simulink model "speed_controller_Harness1"  (R2020b)
settings: Solver=FixedStepDiscrete  StartTime=0.0  StopTime=500  FixedStep=double(Ts)  RelTol=1e-3
settings Model: DataDictionary=speed_controller.sldd  Creator=Dmitry  LastModifiedBy=Dmitry

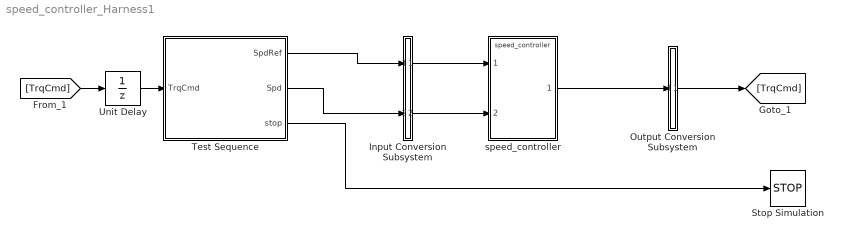
== system speed_controller_Harness1 ==
  Input Conversion Subsystem : Subsystem  Tag=__SLT_ICS__  Description=|
      | Signal spec.
      | and routing
      settings: AttributesFormatString=%<Description>
  Output Conversion Subsystem : Subsystem  Tag=__SLT_OCS__  Description=|
      | Signal spec.
      | and routing
      settings: AttributesFormatString=%<Description>
  Stop Simulation : Stop
  Test Sequence : Test Sequence  TreatAsAtomicUnit=on
  Unit Delay : UnitDelay  SampleTime=-1  HasFrameUpgradeWarning=on
  speed_controller : ModelReference  ModelNameDialog=speed_controller  SimulationMode=Normal  ModelReferenceVersion=1.4
  wires:
  Test Sequence/1(SpdRef) -> Input Conversion Subsystem/1(Inport_1)
  Test Sequence/2(Spd) -> Input Conversion Subsystem/2(Inport_2)
  [TrqCmd] -> Unit Delay/1
  Output Conversion Subsystem/1(Outport_1) -> [TrqCmd]
  Input Conversion Subsystem/1(Outport_1) -> speed_controller/1
  Input Conversion Subsystem/2(Outport_2) -> speed_controller/2
  speed_controller/1 -> Output Conversion Subsystem/1(Inport_1)
  Unit Delay/1 -> Test Sequence/1(TrqCmd)
  Test Sequence/3(stop) -> Stop Simulation/1

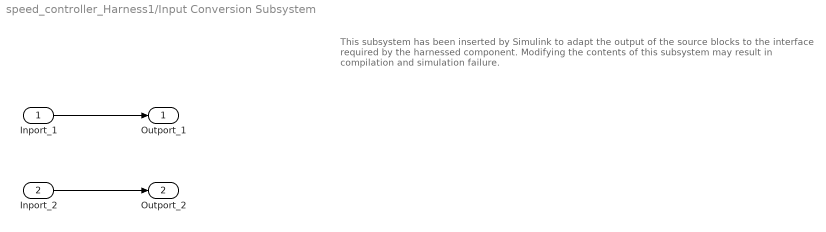
== system speed_controller_Harness1/Input Conversion Subsystem ==
  note: This subsystem has been inserted by Simulink to adapt the output of the source blocks to the interface required by the harnessed component.
      |  Modifying the contents of this subsystem may result in compilation and simulation failure.
  Inport_1 : Inport
  Inport_2 : Inport  Port=2
  Outport_1 : Outport
  Outport_2 : Outport  Port=2
  wires:
  Inport_1/1 -> Outport_1/1
  Inport_2/1 -> Outport_2/1

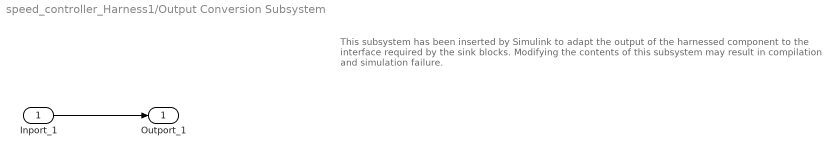
== system speed_controller_Harness1/Output Conversion Subsystem ==
  note: This subsystem has been inserted by Simulink to adapt the output of the harnessed component to the interface required by the sink blocks.
      |  Modifying the contents of this subsystem may result in compilation and simulation failure.
  Inport_1 : Inport
  Outport_1 : Outport
  wires:
  Inport_1/1 -> Outport_1/1

== stateflow chart speed_controller_Harness1/Test Sequence ==
  settings: stateMachineType=SIMPLIFIED_MACHINE
  state step_1
    %% Initialize data outputs.
    SpdRef = 0;
    Spd = 0;
  state check_1
    assert(abs(TrqCmd)<eps,'step 1: torque command is not zero');
  state step_2
    Spd=1;
  state check_2
    assert(TrqCmd<0,'step 2: torque command is not zero');
  state stop
    stop=true;
  (default) -> step_1
  step_1 -> check_1 : [
      | after(100,msec)
      | ]
  check_1 -> step_2 : [
      | true
      | ]
  step_2 -> check_2 : [
      | after(100,msec)
      | ]
  check_2 -> stop : [
      | true
      | ]
  data: TrqCmd input single size=[1]; SpdRef output single size=[1]; Spd output single size=[1]; eps constant single =1e-6; stop output boolean =false
